simulink model "landing_gear_forces_and_moments_example"  (R2022a)
settings: Solver=ode4  StartTime=0.0  StopTime=60  FixedStep=1e-4  RelTol=1e-3
undefined symbols (not defined in the file or in its folder): Earth, WGS84
libraries: simulink_extras x2, aerolib6dof2 x1, aerolibtransform2 x1
settings Model: Creator=kboychev  LastModifiedBy=Kiril Boychev
settings SolverCC: AlgebraicLoopSolver=TrustRegion
settings DataIOCC: ReturnWorkspaceOutputs=off
settings DebuggingCC: UnconnectedInputMsg=warning  UnconnectedOutputMsg=warning  UnconnectedLineMsg=warning  SFMachineParentedDataDiag=warning  ArithmeticOperatorsInVariantConditions=warning
settings SFSimCC: CustomCodeUndefinedFunction=UseInterfaceOnly

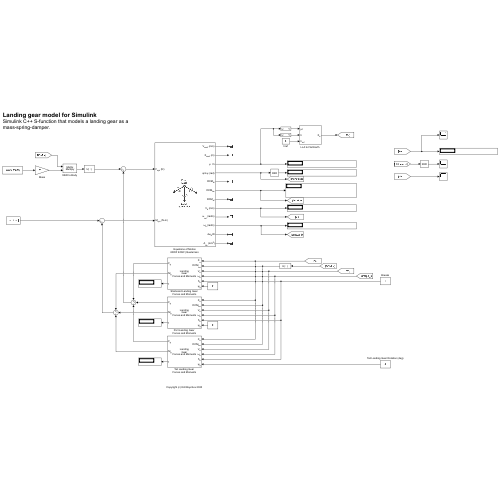
[thumbnail: Simulink's stored preview of the top-level diagram]
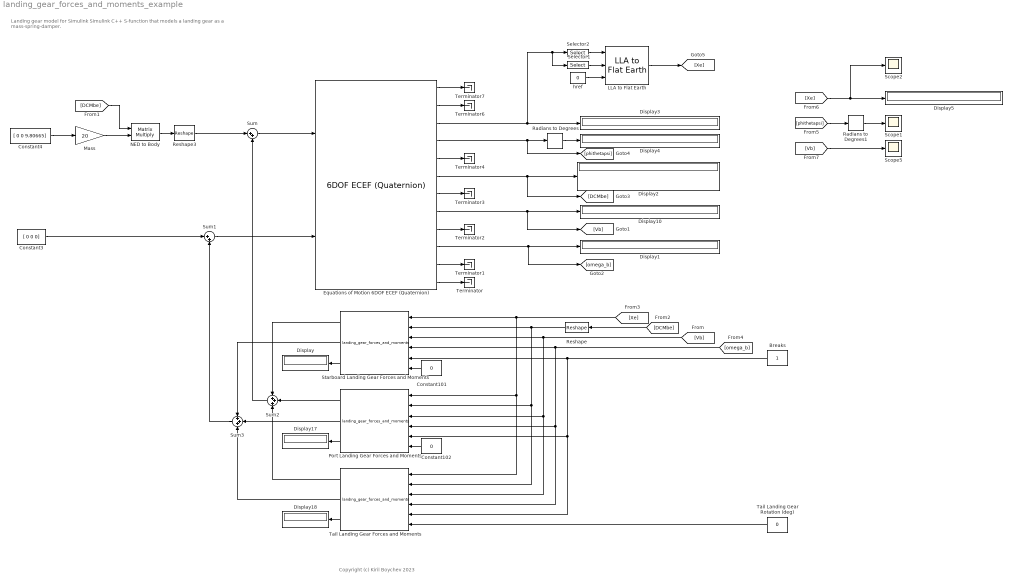
== system landing_gear_forces_and_moments_example ==
  note: Copyright (c) Kiril Boychev 2023
  note: Landing gear model for Simulink
      | Simulink C++ S-function that models a landing gear as a mass-spring-damper.
  Breaks : Constant
  Constant101 : Constant  Value=0
  Constant102 : Constant  Value=0
  Constant3 : Constant  Value=[ 0 0 0]
  Constant4 : Constant  Value=[ 0 0 9.80665]
  Display{,1..5,10,17..18} (9 alike) : Display
  Equations of Motion 6DOF ECEF (Quaternion) : aerolib6dof2/6DOF ECEF (Quaternion)  units=Metric (MKS)  mtype=Fixed  xg_0=[ 0 0 0.5]  Vm_0=[0 0 0]  eul_0=[0 0 0]  pm_0=[0 0 0]  mass_0=20  mass_e=0.5  mass_f=2.0  inertia=|  inertia_e=eye(3)  inertia_f=2*eye(3)  vre_flag=on  abi_flag=off  ptype=Earth (WGS84)  R=6378137  F=1/298.257223563  w_E=7292115e-11  angle_in=Internal  LG0=0  quat_statename=''  pm_statename=''  Vm_statename=''  posECEF_statename=''  posECI_statename=''  LG_statename=''  mass_statename=''
      | [    6.2710   -0.0004    0.2725;
      |    -0.0004    3.5260         0;
      |     0.2725         0    9.6700]
      settings: SourceProductBaseCode=AE
  "LLA to Flat Earth " : aerolibtransform2/LLA to Flat Earth  units=Metric (MKS)  ptype=Earth (WGS84)  F=1/298.257223563  R=6378137  refPosPort=off  LL0=[0 0]  psi=0
      settings: SourceProductBaseCode=AE
  Mass : Gain  Gain=20  SaturateOnIntegerOverflow=on  OutDataTypeStr=Inherit: Same as input  ParamDataTypeStr=Inherit: Same as input
  NED to Body : Product  Multiplication=Matrix(*)  InputSameDT=on  SaturateOnIntegerOverflow=on  OutDataTypeStr=Inherit: Same as first input
  Port Landing Gear Forces and Moments : S-Function  FunctionName=landing_gear_forces_and_moments  Parameters=Xcg,Xg,dz_max,k,c,mus,mud,mur  SFunctionDeploymentMode=off  EnableBusSupport=off  mask(Landing gear forces and moments){Xcg=[0 0 0], Xg=[ 1 -0.5 0.5], dz_max=0.03, k=6.5378e+04, c=2.2870e+03, mus=1.2, mud=1.1, mur=0.02}
      mask prompts: Xcg "Centre of gravity position"; Xg "Landing gear position"; dz_max "Landing gear maximum compression length"; k "Stiffness coefficient"; c "Damping coefficient"; mus "Static friction coefficient"; mud "Dynamic friction coefficient"; mur "Rolling friction coefficient"
      mask help: Landing gear forces and moments are caclulated from the following equations: Fn=-k*f*dz_max-c*Vz, M=cross(Xg,F) where k is the stiffness coefficient, f is the compression ratio, dz_max is the maximum compression length, c is the damping coefficient, Vz is the landing gear velocity along the z-axis of the body-fixed coordinate frame, Xg is the compressed gear vector, and F is the total force from the gear including friction. An initial values for the stiffness coefficients can be obtained from the following equations: k=(1/dz_max)*W*10 and c=2*sqrt(k*m) where W and m are the aircraft weight and mass.
      mask Display:
      | fprintf('Landing\nGear\nForces and Moments');
      | port_label('input', 1, 'X_{e}','texmode','on');
      | port_label('input', 2, 'DCM_{be}','texmode','on');
      | port_label('input', 3, 'V_{b}','texmode','on');
      | port_label('input', 4, '\omega_{b}','texmode','on');
      | port_label('input', 5, '\delta_{b}','texmode','on');
      | port_label('input', 6, '\psi_{g}','texmode','on');
      | port_label('output', 1, 'F_{g}','texmode','on');
      | port_label('output', 2, 'M_{g}','texmode','on');
      | port_label('output', 3, 'f','texmode','on');
  Radians to Degrees : simulink_extras/Transformations/Radians to Degrees
  Radians to Degrees1 : simulink_extras/Transformations/Radians to Degrees
  Reshape : Reshape
  Reshape3 : Reshape
  Scope1 : Scope
  Scope2 : Scope
  Scope5 : Scope
  Selector1 : Selector  IndexMode=Zero-based  InputPortWidth=3  IndexOptions=Starting index (dialog)  Indices=2  OutputSizes=1
  Selector2 : Selector  IndexMode=Zero-based  InputPortWidth=3  IndexOptions=Index vector (dialog)  Indices=[ 0 1 ]  OutputSizes=1
  Starboard Landing Gear Forces and Moments : S-Function  FunctionName=landing_gear_forces_and_moments  Parameters=Xcg,Xg,dz_max,k,c,mus,mud,mur  SFunctionDeploymentMode=off  EnableBusSupport=off  mask(Landing gear forces and moments){Xcg=[0 0 0], Xg=[ 1 0.5 0.5], dz_max=0.03, k=6.5378e+04, c=2.2870e+03, mus=1.2, mud=1.1, mur=0.02}
      mask prompts: Xcg "Centre of gravity position"; Xg "Landing gear position"; dz_max "Landing gear maximum compression length"; k "Stiffness coefficient"; c "Damping coefficient"; mus "Static friction coefficient"; mud "Dynamic friction coefficient"; mur "Rolling friction coefficient"
      mask help: Landing gear forces and moments are caclulated from the following equations: Fn=-k*f*dz_max-c*Vz, M=cross(Xg,F) where k is the stiffness coefficient, f is the compression ratio, dz_max is the maximum compression length, c is the damping coefficient, Vz is the landing gear velocity along the z-axis of the body-fixed coordinate frame, Xg is the compressed gear vector, and F is the total force from the gear including friction. An initial values for the stiffness coefficients can be obtained from the following equations: k=(1/dz_max)*W*10 and c=2*sqrt(k*m) where W and m are the aircraft weight and mass.
      mask Display:
      | fprintf('Landing\nGear\nForces and Moments');
      | port_label('input', 1, 'X_{e}','texmode','on');
      | port_label('input', 2, 'DCM_{be}','texmode','on');
      | port_label('input', 3, 'V_{b}','texmode','on');
      | port_label('input', 4, '\omega_{b}','texmode','on');
      | port_label('input', 5, '\delta_{b}','texmode','on');
      | port_label('input', 6, '\psi_{g}','texmode','on');
      | port_label('output', 1, 'F_{g}','texmode','on');
      | port_label('output', 2, 'M_{g}','texmode','on');
      | port_label('output', 3, 'f','texmode','on');
  Sum : Sum  Inputs=|++
  Sum1 : Sum  Inputs=|++
  Sum2 : Sum  Inputs=+++
  Sum3 : Sum  Inputs=+++
  Tail Landing Gear Forces and Moments : S-Function  FunctionName=landing_gear_forces_and_moments  Parameters=Xcg,Xg,dz_max,k,c,mus,mud,mur  SFunctionDeploymentMode=off  EnableBusSupport=off  mask(Landing gear forces and moments){Xcg=[0 0 0], Xg=[ -2 0 0.25], dz_max=0.01, k=196133, c=3.9611e+03, mus=1.6, mud=1.3, mur=0.02}
      mask prompts: Xcg "Centre of gravity position"; Xg "Landing gear position"; dz_max "Landing gear maximum compression length"; k "Stiffness coefficient"; c "Damping coefficient"; mus "Static friction coefficient"; mud "Dynamic friction coefficient"; mur "Rolling friction coefficient"
      mask help: Landing gear forces and moments are caclulated from the following equations: Fn=-k*f*dz_max-c*Vz, M=cross(Xg,F) where k is the stiffness coefficient, f is the compression ratio, dz_max is the maximum compression length, c is the damping coefficient, Vz is the landing gear velocity along the z-axis of the body-fixed coordinate frame, Xg is the compressed gear vector, and F is the total force from the gear including friction. An initial values for the stiffness coefficients can be obtained from the following equations: k=(1/dz_max)*W*10 and c=2*sqrt(k*m) where W and m are the aircraft weight and mass.
      mask Display:
      | fprintf('Landing\nGear\nForces and Moments');
      | port_label('input', 1, 'X_{e}','texmode','on');
      | port_label('input', 2, 'DCM_{be}','texmode','on');
      | port_label('input', 3, 'V_{b}','texmode','on');
      | port_label('input', 4, '\omega_{b}','texmode','on');
      | port_label('input', 5, '\delta_{b}','texmode','on');
      | port_label('input', 6, '\psi_{g}','texmode','on');
      | port_label('output', 1, 'F_{g}','texmode','on');
      | port_label('output', 2, 'M_{g}','texmode','on');
      | port_label('output', 3, 'f','texmode','on');
  Tail Landing Gear Rotation (deg) : Constant  Value=0
  Terminator{,1..4,6..7} (7 alike) : Terminator
  href : Constant  Value=0
  wires:
  Equations of Motion 6DOF ECEF (Quaternion)/3 -> Selector1/1, Selector2/1, Display3/1
  Selector1/1 -> "LLA to Flat Earth "/2
  Selector2/1 -> "LLA to Flat Earth "/1
  href/1 -> "LLA to Flat Earth "/3
  Equations of Motion 6DOF ECEF (Quaternion)/8 -> [Vb], Display10/1
  Equations of Motion 6DOF ECEF (Quaternion)/10 -> [omega_b], Display1/1
  Equations of Motion 6DOF ECEF (Quaternion)/6 -> [DCMbe], Display2/1
  Equations of Motion 6DOF ECEF (Quaternion)/12 -> Terminator/1
  Equations of Motion 6DOF ECEF (Quaternion)/11 -> Terminator1/1
  Equations of Motion 6DOF ECEF (Quaternion)/9 -> Terminator2/1
  Equations of Motion 6DOF ECEF (Quaternion)/7 -> Terminator3/1
  Equations of Motion 6DOF ECEF (Quaternion)/5 -> Terminator4/1
  Equations of Motion 6DOF ECEF (Quaternion)/4 -> [phithetapsi], Radians to Degrees/1
  Equations of Motion 6DOF ECEF (Quaternion)/2 -> Terminator6/1
  Equations of Motion 6DOF ECEF (Quaternion)/1 -> Terminator7/1
  Sum1/1 -> Equations of Motion 6DOF ECEF (Quaternion)/2
  Constant4/1 -> Mass/1
  Constant3/1 -> Sum1/1
  "LLA to Flat Earth "/1 -> [Xe]
  Radians to Degrees/1 -> Display4/1
  Starboard Landing Gear Forces and Moments/1 -> Sum2/1
  Tail Landing Gear Forces and Moments/1 -> Sum2/3
  Port Landing Gear Forces and Moments/2 -> Sum3/2
  Starboard Landing Gear Forces and Moments/2 -> Sum3/1
  Tail Landing Gear Forces and Moments/2 -> Sum3/3
  Breaks/1 -> Tail Landing Gear Forces and Moments/5, Port Landing Gear Forces and Moments/5, Starboard Landing Gear Forces and Moments/5
  Mass/1 -> NED to Body/2
  NED to Body/1 -> Reshape3/1
  [DCMbe] -> NED to Body/1
  Reshape/1 -> Tail Landing Gear Forces and Moments/2, Port Landing Gear Forces and Moments/2, Starboard Landing Gear Forces and Moments/2
  [Vb] -> Tail Landing Gear Forces and Moments/3, Port Landing Gear Forces and Moments/3, Starboard Landing Gear Forces and Moments/3
  [omega_b] -> Tail Landing Gear Forces and Moments/4, Port Landing Gear Forces and Moments/4, Starboard Landing Gear Forces and Moments/4
  [phithetapsi] -> Radians to Degrees1/1
  [Xe] -> Scope2/1, Display5/1
  Radians to Degrees1/1 -> Scope1/1
  Port Landing Gear Forces and Moments/1 -> Sum2/2
  [Xe] -> Starboard Landing Gear Forces and Moments/1, Tail Landing Gear Forces and Moments/1, Port Landing Gear Forces and Moments/1
  [DCMbe] -> Reshape/1
  Starboard Landing Gear Forces and Moments/3 -> Display/1
  Port Landing Gear Forces and Moments/3 -> Display17/1
  Tail Landing Gear Forces and Moments/3 -> Display18/1
  Sum3/1 -> Sum1/2
  Sum/1 -> Equations of Motion 6DOF ECEF (Quaternion)/1
  Constant101/1 -> Starboard Landing Gear Forces and Moments/6
  Constant102/1 -> Port Landing Gear Forces and Moments/6
  [Vb] -> Scope5/1
  Sum2/1 -> Sum/2
  Tail Landing Gear Rotation (deg)/1 -> Tail Landing Gear Forces and Moments/6
  Reshape3/1 -> Sum/1
